simulink model "questao01_well"  (R2020a)
settings: Solver=VariableStepAuto  StartTime=0.0  StopTime=90  RelTol=1e-3
values from neighbouring files (symbols this model uses):
  A = [1 2 0;-1 -1 -1;0 2 -1]    [lqr_estudos.m]    (also in questao2_pat.m = [1 2 0; -1 -1 -1; 0 2 -1])
  B = [0;0;2]    [lqr_estudos.m]    (also in questao2_pat.m)
  C = [0 1 0;0 0 1]    [lqr_estudos.m]    (also in questao2_pat.m = [0 1 0; 0 0 1])
  d_i = 1    [questao1_well.m]
  K = Kbar*CMbar*inv(CM)    [estudos_versao_laurinda.m]    (also in lqr_estudos.m = lqr(A,B,Q,R); questao1_pat.m = Ka(1:3); questao1_well.m = Ka(1:3); questao2_pat.m = place(A,B,newpoles))
  Kz = Ka(4)    [questao1_pat.m]    (also in questao1_well.m)
settings Model: Creator=wwagner  LastModifiedBy=wwagner

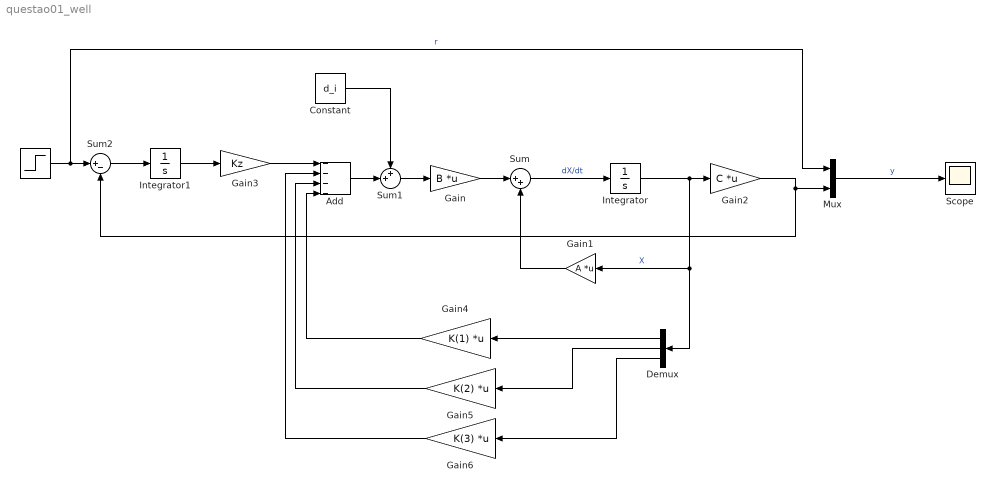
== system questao01_well ==
  " " : Step  Tag=r  SampleTime=0
  Add : Sum  Inputs=----
  Constant : Constant  Value=d_i
  Demux : Demux  Outputs=3
  Gain : Gain  Gain=B  Multiplication=Matrix(K*u)
  Gain1 : Gain  Gain=A  Multiplication=Matrix(K*u)
  Gain2 : Gain  Gain=C  Multiplication=Matrix(K*u)
  Gain3 : Gain  Gain=Kz
  Gain4 : Gain  Gain=K(1)  Multiplication=Matrix(K*u)
  Gain5 : Gain  Gain=K(2)  Multiplication=Matrix(K*u)
  Gain6 : Gain  Gain=K(3)  Multiplication=Matrix(K*u)
  Integrator : Integrator
  Integrator1 : Integrator
  Mux : Mux  Inputs=2
  Scope : Scope
  Sum : Sum  Inputs=|++
  Sum1 : Sum  Inputs=++|
  Sum2 : Sum  Inputs=|+-
  wires:
  Integrator/1 -> Demux/1, Gain1/1, Gain2/1  "X"
  Gain/1 -> Sum/1
  Gain1/1 -> Sum/2
  Sum/1 -> Integrator/1  "dX/dt"
  Gain2/1 -> Mux/2, Sum2/2
  Mux/1 -> Scope/1  "y"
  Sum2/1 -> Integrator1/1
  " "/1 -> Sum2/1, Mux/1  "r"
  Integrator1/1 -> Gain3/1
  Demux/1 -> Gain4/1
  Demux/2 -> Gain5/1
  Demux/3 -> Gain6/1
  Gain3/1 -> Add/1
  Gain4/1 -> Add/4
  Gain5/1 -> Add/3
  Gain6/1 -> Add/2
  Sum1/1 -> Gain/1
  Add/1 -> Sum1/2
  Constant/1 -> Sum1/1
